simulink model "spring_damper"  (R2025b)
settings: Solver=VariableStepAuto  StartTime=0.0  StopTime=30.0  MaxStep=0.01  RelTol=1e-3
settings Model: Creator=Sathsara  LastModifiedBy=Sathsara

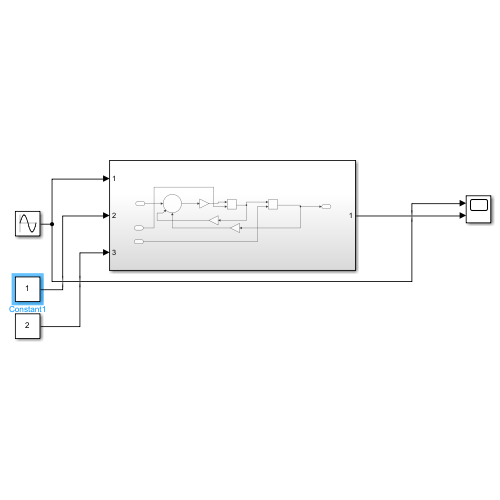
[thumbnail: Simulink's stored preview of the top-level diagram]
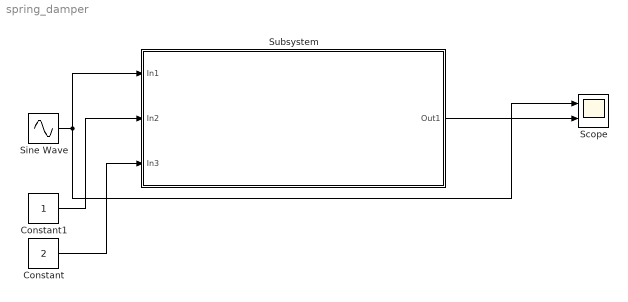
== system spring_damper ==
  Constant : Constant  Value=2
  Constant1 : Constant
  Scope : Scope  NumInputPorts=2
      settings: ActiveDisplayYMinimum=-2.5528936295620492  ActiveDisplayYMaximum=2.9760580521084568
  Sine Wave : Sin  Amplitude=2  Frequency=2  SampleTime=0
  Subsystem : Subsystem
  wires:
  Sine Wave/1 -> Subsystem/1(In1), Scope/1
  Constant1/1 -> Subsystem/2(In2)
  Constant/1 -> Subsystem/3(In3)
  Subsystem/1(Out1) -> Scope/2

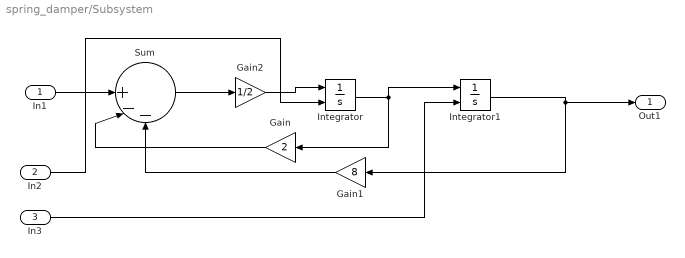
== system spring_damper/Subsystem ==
  In1 : Inport
  In2 : Inport  Port=2
  In3 : Inport  Port=3
  Gain : Gain  Gain=2
  Gain1 : Gain  Gain=8
  Gain2 : Gain  Gain=1/2
  Integrator : Integrator  InitialConditionSource=external  InitialCondition=2
  Integrator1 : Integrator  InitialConditionSource=external  InitialCondition=1
  Sum : Sum  Inputs=||+--
  Out1 : Outport
  wires:
  Integrator1/1 -> Out1/1, Gain1/1
  Sum/1 -> Gain2/1
  In1/1 -> Sum/1
  Integrator/1 -> Integrator1/1, Gain/1
  Gain1/1 -> Sum/3
  Gain/1 -> Sum/2
  Gain2/1 -> Integrator/1
  In2/1 -> Integrator/2
  In3/1 -> Integrator1/2
